simulink model "Controller_Tank_2_Primitives"  (R2012b)
settings: Solver=FixedStepDiscrete  StartTime=0.0  StopTime=10.0  FixedStep=0.1  RelTol=1e-3
libraries: simulink x6
settings Model: Creator=Kerianne  LastModifiedBy=Kerianne
settings DataIOCC: SaveFormat=Structure
settings OptimizationCC: InlineParams=on

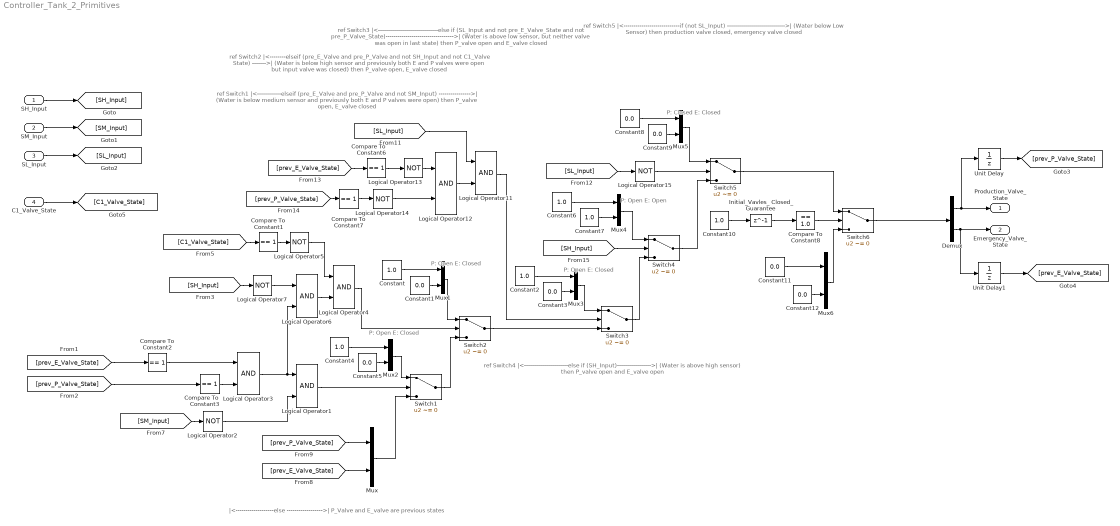
== system Controller_Tank_2_Primitives ==
  note: P: Open
      | E: Closed
  note: P: Open
      | E: Closed
  note: P: Open
      | E: Closed
  note: P: Open
      | E: Open
  note: P: Closed
      | E: Closed
  note: ref Switch5
      | |<----------------------------if (not SL_Input) ----------------------------->|
      | (Water below Low Sensor)
      | then production valve closed, emergency valve closed
  note: ref Switch3
      | |<------------------------------else if (SL_Input and not pre_E_Valve_State and not pre_P_Valve_State)---------------------------------->|
      | (Water is above low sensor, but neither valve was open in last state)
      | then P_valve open and E_valve closed
  note: ref Switch2
      | |<--------elseif (pre_E_Valve and pre_P_Valve and not SH_Input and not C1_Valve State) ------->|
      | (Water is below high sensor  and previously both E and P valves were open but input valve was closed)
      | then P_valve open, E_valve closed
  note: ref Switch4
      | |<----------------------else if (SH_Input)----------------->|
      | (Water is above high sensor)
      | then P_valve open and E_valve open
  note: ref Switch1
      | |<------------elseif (pre_E_Valve and pre_P_Valve and not SM_Input) ---------------->|
      | (Water is below medium sensor and previously both E and P valves were open)
      | then P_valve open, E_valve closed
  note: |<-------------------else ------------------>|
      | P_Valve and E_valve are previous states
  SH_Input : Inport  OutDataTypeStr=double
  SM_Input : Inport  Port=2  OutDataTypeStr=double
  SL_Input : Inport  Port=3  OutDataTypeStr=double
  C1_Valve_State : Inport  Port=4  OutDataTypeStr=double
  Compare To Constant{1..3,6..7} (5 alike) : simulink/Logic and Bit Operations/Compare To Constant  relop===  const=1  OutDataTypeStr=boolean
  Compare To Constant8 : simulink/Logic and Bit Operations/Compare To Constant  relop===  const=1.0  OutDataTypeStr=boolean
  Constant{,2,4,6..7,10} (6 alike) : Constant  Value=1.0
  Constant{1,3,5,8..9,11..12} (7 alike) : Constant  Value=0.0
  Demux : Demux  Outputs=2
  Initial_Vavles_ Closed_Guarantee : Delay  DelayLength=1
  Logical Operator{1,3..4,6,11..12} (6 alike) : Logic  AllPortsSameDT=off  OutDataTypeStr=boolean
  Logical Operator{2,5,7,13..15} (6 alike) : Logic  Operator=NOT  AllPortsSameDT=off  OutDataTypeStr=boolean
  Mux{,1..6} (7 alike) : Mux  Inputs=2
  Switch{1..6} (6 alike) : Switch  Criteria=u2 ~= 0
  Unit Delay : UnitDelay  SampleTime=-1
  Unit Delay1 : UnitDelay  SampleTime=-1
  Production_Valve_State : Outport
  Emergency_Valve_State : Outport  Port=2
  wires:
  SH_Input/1 -> [SH_Input]
  SL_Input/1 -> [SL_Input]
  SM_Input/1 -> [SM_Input]
  C1_Valve_State/1 -> [C1_Valve_State]
  [prev_P_Valve_State] -> Mux/1
  [prev_E_Valve_State] -> Mux/2
  Mux/1 -> Switch1/3
  Constant/1 -> Mux1/1
  Constant1/1 -> Mux1/2
  Logical Operator1/1 -> Switch1/2
  [SM_Input] -> Logical Operator2/1
  Switch1/1 -> Switch2/3
  Logical Operator4/1 -> Switch2/2
  Mux1/1 -> Switch2/1
  [prev_E_Valve_State] -> Compare To Constant2/1
  [prev_P_Valve_State] -> Compare To Constant3/1
  [C1_Valve_State] -> Compare To Constant1/1
  Logical Operator5/1 -> Logical Operator4/1
  Logical Operator6/1 -> Logical Operator4/2
  Logical Operator3/1 -> Logical Operator6/2, Logical Operator1/1
  Logical Operator2/1 -> Logical Operator1/2
  [SH_Input] -> Logical Operator7/1
  Logical Operator7/1 -> Logical Operator6/1
  Constant4/1 -> Mux2/1
  Constant5/1 -> Mux2/2
  Mux2/1 -> Switch1/1
  Constant2/1 -> Mux3/1
  Constant3/1 -> Mux3/2
  Mux3/1 -> Switch3/1
  [prev_E_Valve_State] -> Compare To Constant6/1
  [prev_P_Valve_State] -> Compare To Constant7/1
  Logical Operator13/1 -> Logical Operator12/1
  Logical Operator12/1 -> Logical Operator11/2
  [SL_Input] -> Logical Operator11/1
  Logical Operator14/1 -> Logical Operator12/2
  Constant6/1 -> Mux4/1
  Constant7/1 -> Mux4/2
  Mux4/1 -> Switch4/1
  Logical Operator15/1 -> Switch5/2
  [SL_Input] -> Logical Operator15/1
  Constant8/1 -> Mux5/1
  Constant9/1 -> Mux5/2
  Mux5/1 -> Switch5/1
  Compare To Constant1/1 -> Logical Operator5/1
  Compare To Constant2/1 -> Logical Operator3/1
  Compare To Constant3/1 -> Logical Operator3/2
  Compare To Constant6/1 -> Logical Operator13/1
  Compare To Constant7/1 -> Logical Operator14/1
  Constant10/1 -> Initial_Vavles_ Closed_Guarantee/1
  Initial_Vavles_ Closed_Guarantee/1 -> Compare To Constant8/1
  Compare To Constant8/1 -> Switch6/2
  Constant11/1 -> Mux6/1
  Constant12/1 -> Mux6/2
  Switch5/1 -> Switch6/1
  Mux6/1 -> Switch6/3
  Switch6/1 -> Demux/1
  [SH_Input] -> Switch4/2
  Logical Operator11/1 -> Switch3/2
  Switch2/1 -> Switch3/3
  Switch3/1 -> Switch4/3
  Switch4/1 -> Switch5/3
  Demux/2 -> Emergency_Valve_State/1, Unit Delay1/1
  Demux/1 -> Unit Delay/1, Production_Valve_State/1
  Unit Delay/1 -> [prev_P_Valve_State]
  Unit Delay1/1 -> [prev_E_Valve_State]
